simulink model "sampleModel1900"  (R2023a)
settings: Solver=VariableStepAuto  StartTime=0.0  StopTime=10.0  RelTol=1e-3
libraries: hdlsllib x2, simulink x1
settings Model: Creator=user1  LastModifiedBy=user1

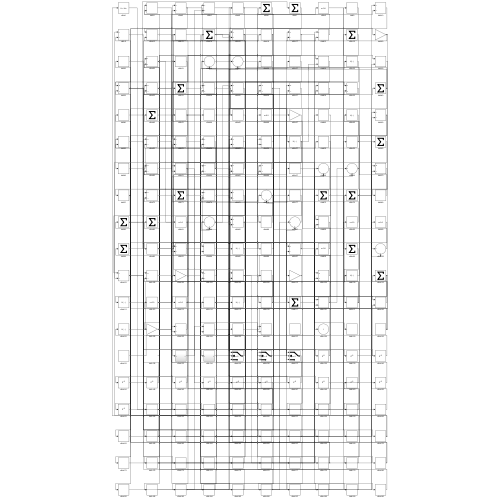
[thumbnail: Simulink's stored preview of the top-level diagram]
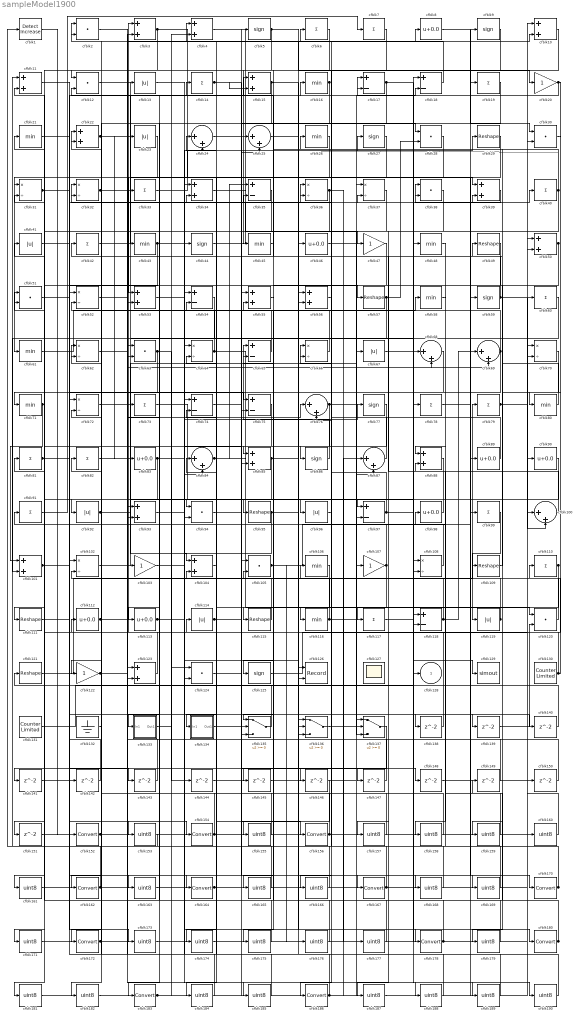
== system sampleModel1900 ==
  cfblk1 : simulink/Logic and Bit Operations/Detect Increase  vinit=0.0  OutDataTypeStr=boolean
      settings: LibrarySourceBlock=|
      | hdlsllib/Logic and Bit
      | Operations/Detect
      | Increase
  cfblk{3..4,10..11,15,22,34,39,50,53,55..56,85,88,93,101,104,123} (18 alike) : Sum
  cfblk{24..25,68..69,76,84,87,100} (8 alike) : Sum  Inputs=|++
  cfblk{31..32,36..37,52,62,64,66,70,72,102,108} (12 alike) : Product  Inputs=*/  RndMeth=Zero  SaturateOnIntegerOverflow=on
  cfblk{20,47,103,107,122} (5 alike) : Gain
  cfblk{2,12,28,30,38,51,63,94,105,120,124} (11 alike) : DotProduct  OutDataTypeStr=Inherit: Inherit via internal rule
  cfblk{16,21,26,43,45,48,58,61,71,80,106,116} (12 alike) : MinMax
  cfblk{29,49,57,95,109,111,115,121} (8 alike) : Reshape
  cfblk{6..7,14,19,33,40,42,60,73,78..79,81..82,91,99,110,117} (17 alike) : Sum  Inputs=+
  cfblk{8,46,83,89..90,98,112..113} (8 alike) : Bias  Bias=0.0  SaturateOnIntegerOverflow=off
  cfblk{13,23,41,67,92,96,114,119} (8 alike) : Abs  SaturateOnIntegerOverflow=off
  cfblk{17..18,35,54,65,74..75,97,118} (9 alike) : Sum  Inputs=+-
  cfblk{5,9,27,44,59,77,86,125} (8 alike) : Signum
  cfblk126 : Record  FileSettingsInternal="{\"entries\":[{\"content\":{\"excelSettings\":{\"content\":{},\"type\":\"Streamout.ExcelSettings\"}},\"type\":\"Streamout.FileSettingStorage\",\"uuid\":\"\"}],\"packageUris\":[\"http:\\/\\/schema.mathworks.com\\/mf0\\/streamout_blocks\\/R2020a\"],\"version\":\"1.0\"}"  Layout=[1 1]  SignalsInternal="{\"entries\":[{\"content\":{\"signals\":[{\"content\":{\"blockPath\":[],\"dimensions\":[1],\"domain\":\"\",\"lineColor\":\"#a2142f\",\"plots\":[1],\"port\":1,\"signalID\":4952,\"signalName\":\"XY Graph:1\"},\"type\":\"RecordBlkView.Signal\",\"uuid\":\"\"},{\"content\":{\"blockPath\":[],\"dimensions\":[1],\"domain\":\"\",\"lineColor\":\"#139fff\",\"plots\":[1],\"port\":2,\"signalID\":4955,\"signalName\":\"XY Graph:2\"},\"type\":\"RecordBlkView.Signal\",\"uuid\":\"\"}]},\"type\":\"RecordBlkView.InputSignals\",\"uuid\":\"\"}],\"packageUris\":[\"http:\\/\\/schema.mathworks.com\\/mf0\\/streamout_blocks\\/R2020a\"],\"version\":\"1.0\"}"  VisualizationBindings="{\"xyplotplugin\":{\"info\":[{\"series\":[{\"bindingParametersList\":[{\"parameter\":\"X-Axis\",\"signalID\":4952,\"signalName\":\"XY Graph:1\"},{\"parameter\":\"Y-Axis\",\"signalID\":4955,\"signalName\":\"XY Graph:2\"}],\"seriesID\":55809}],\"subplotID\":1}]}}"  CompatibilityTag=XY  st=-1
  cfblk127 : Scope
      settings: Floating=on
  cfblk129 : ToWorkspace  VariableName=simout  SaveFormat=Timeseries  SampleTime=-1
  cfblk130 : hdlsllib/Sources/Counter Limited  uplimit=7  tsamp=-1
  cfblk131 : hdlsllib/Sources/Counter Limited  uplimit=7  tsamp=-1
  cfblk132 : Ground
  cfblk133 : Subsystem
      settings: LibrarySourceBlock=|
      | hdlsllib/Ports &
      | Subsystems/Subsystem
  cfblk134 : Subsystem
      settings: LibrarySourceBlock=|
      | hdlsllib/Ports &
      | Subsystems/Subsystem
  cfblk135 : Switch  SaturateOnIntegerOverflow=off  InputSameDT=off
  cfblk136 : Switch  SaturateOnIntegerOverflow=off  InputSameDT=off
  cfblk137 : Switch  SaturateOnIntegerOverflow=off  InputSameDT=off
  cfblk{138..151} (14 alike) : Delay  SampleTime=1
  cfblk{152,154,156,162,164,167,170,172,178,180,183,186} (12 alike) : DataTypeConversion  SaturateOnIntegerOverflow=off  RndMeth=Floor
  cfblk{153,155,157..161,163,165..166,168..169,171,173..177,179,181..182,184..185,187..190} (27 alike) : DataTypeConversion  OutDataTypeStr=uint8  SaturateOnIntegerOverflow=off  RndMeth=Floor
  cfblk128 : Outport  VectorParamsAs1DForOutWhenUnconnected=off
  wires:
  cfblk108/1 -> cfblk91/1
  cfblk123/1 -> cfblk3/1
  cfblk58/1 -> cfblk117/1
  cfblk98/1 -> cfblk94/1
  cfblk84/1 -> cfblk120/1, cfblk35/1
  cfblk120/1 -> cfblk79/1
  cfblk86/1 -> cfblk65/1
  cfblk100/1 -> cfblk42/1
  cfblk73/1 -> cfblk96/1
  cfblk71/1 -> cfblk101/1, cfblk51/2
  cfblk91/1 -> cfblk7/1
  cfblk12/1 -> cfblk39/1
  cfblk32/1 -> cfblk104/1, cfblk75/1
  cfblk30/1 -> cfblk114/1
  cfblk110/1 -> cfblk118/2, cfblk157/1
  cfblk27/1 -> cfblk95/1
  cfblk118/1 -> cfblk84/1, cfblk69/1
  cfblk40/1 -> cfblk116/1, cfblk24/2, cfblk12/2
  cfblk42/1 -> cfblk16/1
  cfblk99/1 -> cfblk119/1
  cfblk82/1 -> cfblk154/1
  cfblk132/1 -> cfblk22/1
  cfblk74/1 -> cfblk156/1
  cfblk121/1 -> cfblk109/1
  cfblk54/1 -> cfblk183/1
  cfblk115/1 -> cfblk13/1
  cfblk26/1 -> cfblk134/1(In1)
  cfblk63/1 -> cfblk71/1, cfblk144/1
  cfblk105/1 -> cfblk9/1, cfblk176/1
  cfblk2/1 -> cfblk63/2
  cfblk75/1 -> cfblk133/1(In1)
  cfblk69/1 -> cfblk135/1, cfblk32/2
  cfblk18/1 -> cfblk6/1
  cfblk113/1 -> cfblk77/1, cfblk126/2
  cfblk44/1 -> cfblk38/1
  cfblk57/1 -> cfblk101/2, cfblk28/2, cfblk146/1
  cfblk17/1 -> cfblk128/1, cfblk33/1
  cfblk7/1 -> cfblk86/1
  cfblk85/1 -> cfblk46/1, cfblk93/2
  cfblk33/1 -> cfblk29/1
  cfblk5/1 -> cfblk20/1, cfblk151/1
  cfblk31/1 -> cfblk56/2, cfblk75/2, cfblk173/1
  cfblk80/1 -> cfblk26/1
  cfblk68/1 -> cfblk172/1
  cfblk4/1 -> cfblk47/1
  cfblk11/1 -> cfblk164/1
  cfblk102/1 -> cfblk34/1
  cfblk60/1 -> cfblk162/1
  cfblk117/1 -> cfblk48/1
  cfblk61/1 -> cfblk58/1
  cfblk133/1(Out1) -> cfblk124/1
  cfblk10/1 -> cfblk45/1
  cfblk15/1 -> cfblk92/1, cfblk57/1, cfblk125/1
  cfblk56/1 -> cfblk36/1
  cfblk122/1 -> cfblk40/1, cfblk69/2
  cfblk64/1 -> cfblk108/1, cfblk53/2
  cfblk23/1 -> cfblk61/1
  cfblk90/1 -> cfblk123/2
  cfblk22/1 -> cfblk118/1, cfblk83/1
  cfblk95/1 -> cfblk124/2, cfblk10/2
  cfblk1/1 -> cfblk152/1
  cfblk79/1 -> cfblk50/1, cfblk100/2
  cfblk119/1 -> cfblk102/2, cfblk73/1
  cfblk19/1 -> cfblk186/1
  cfblk39/1 -> cfblk38/2
  cfblk136/1 -> cfblk67/1
  cfblk35/1 -> cfblk135/2
  cfblk50/1 -> cfblk115/1, cfblk179/1
  cfblk16/1 -> cfblk113/1, cfblk182/1
  cfblk34/1 -> cfblk107/1
  cfblk37/1 -> cfblk135/3
  cfblk25/1 -> cfblk180/1
  cfblk131/1 -> cfblk108/2
  cfblk89/1 -> cfblk2/1
  cfblk101/1 -> cfblk51/1, cfblk143/1, cfblk163/1
  cfblk36/1 -> cfblk111/1, cfblk177/1
  cfblk65/1 -> cfblk22/2
  cfblk76/1 -> cfblk18/2, cfblk181/1
  cfblk3/1 -> cfblk99/1, cfblk12/1
  cfblk8/1 -> cfblk30/1
  cfblk97/1 -> cfblk129/1, cfblk66/1
  cfblk28/1 -> cfblk53/1
  cfblk46/1 -> cfblk137/1
  cfblk49/1 -> cfblk88/1
  cfblk114/1 -> cfblk136/2, cfblk148/1
  cfblk62/1 -> cfblk23/1
  cfblk111/1 -> cfblk137/2
  cfblk45/1 -> cfblk85/1
  cfblk41/1 -> cfblk17/1
  cfblk96/1 -> cfblk36/2
  cfblk20/1 -> cfblk17/2, cfblk80/1
  cfblk83/1 -> cfblk27/1, cfblk122/1
  cfblk43/1 -> cfblk84/2, cfblk35/2, cfblk171/1
  cfblk87/1 -> cfblk32/1
  cfblk125/1 -> cfblk10/1
  cfblk81/1 -> cfblk37/2, cfblk169/1
  cfblk9/1 -> cfblk31/1
  cfblk59/1 -> cfblk100/1, cfblk15/1
  cfblk51/1 -> cfblk137/3
  cfblk52/1 -> cfblk167/1
  cfblk116/1 -> cfblk39/2, cfblk62/1
  cfblk53/1 -> cfblk85/2
  cfblk66/1 -> cfblk24/1
  cfblk107/1 -> cfblk62/2, cfblk155/1
  cfblk78/1 -> cfblk170/1
  cfblk103/1 -> cfblk178/1
  cfblk109/1 -> cfblk49/1
  cfblk92/1 -> cfblk97/1, cfblk37/1
  cfblk112/1 -> cfblk76/1, cfblk8/1
  cfblk104/1 -> cfblk14/1
  cfblk14/1 -> cfblk15/2, cfblk139/1, cfblk140/1
  cfblk47/1 -> cfblk76/2
  cfblk135/1 -> cfblk41/1
  cfblk130/1 -> cfblk31/2, cfblk4/1, cfblk110/1
  cfblk24/1 -> cfblk28/1
  cfblk94/1 -> cfblk138/1
  cfblk138/1 -> cfblk34/2
  cfblk139/1 -> cfblk120/2
  cfblk140/1 -> cfblk104/2
  cfblk137/1 -> cfblk141/1
  cfblk21/1 -> cfblk142/1
  cfblk142/1 -> cfblk102/1
  cfblk143/1 -> cfblk93/1
  cfblk144/1 -> cfblk97/2
  cfblk29/1 -> cfblk145/1
  cfblk145/1 -> cfblk65/2
  cfblk124/1 -> cfblk147/1
  cfblk147/1 -> cfblk64/2
  cfblk148/1 -> cfblk50/2
  cfblk149/1 -> cfblk56/1
  cfblk150/1 -> cfblk123/1
  cfblk151/1 -> cfblk3/2
  cfblk152/1 -> cfblk136/1, cfblk90/1
  cfblk141/1 -> cfblk153/1
  cfblk153/1 -> cfblk1/1
  cfblk154/1 -> cfblk5/1, cfblk64/1
  cfblk155/1 -> cfblk82/1
  cfblk156/1 -> cfblk105/2, cfblk66/2, cfblk43/1, cfblk59/1
  cfblk157/1 -> cfblk74/1
  cfblk48/1 -> cfblk158/1
  cfblk158/1 -> cfblk74/2
  cfblk70/1 -> cfblk159/1
  cfblk159/1 -> cfblk98/1
  cfblk160/1 -> cfblk70/1
  cfblk88/1 -> cfblk161/1
  cfblk161/1 -> cfblk70/2
  cfblk162/1 -> cfblk94/2, cfblk21/1
  cfblk163/1 -> cfblk60/1
  cfblk164/1 -> cfblk136/3, cfblk89/1
  cfblk6/1 -> cfblk165/1
  cfblk165/1 -> cfblk11/1
  cfblk77/1 -> cfblk166/1
  cfblk166/1 -> cfblk11/2
  cfblk167/1 -> cfblk18/1, cfblk106/1
  cfblk134/1(Out1) -> cfblk168/1
  cfblk168/1 -> cfblk52/1
  cfblk169/1 -> cfblk52/2
  cfblk170/1 -> cfblk88/2, cfblk2/2
  cfblk171/1 -> cfblk78/1
  cfblk172/1 -> cfblk160/1, cfblk44/1
  cfblk173/1 -> cfblk68/1
  cfblk146/1 -> cfblk174/1
  cfblk174/1 -> cfblk68/2
  cfblk55/1 -> cfblk175/1
  cfblk175/1 -> cfblk112/1
  cfblk176/1 -> cfblk55/1
  cfblk177/1 -> cfblk55/2
  cfblk178/1 -> cfblk81/1, cfblk105/1
  cfblk179/1 -> cfblk103/1
  cfblk180/1 -> cfblk149/1, cfblk121/1
  cfblk181/1 -> cfblk25/1
  cfblk182/1 -> cfblk25/2
  cfblk183/1 -> cfblk150/1, cfblk4/2, cfblk87/2
  cfblk106/1 -> cfblk184/1
  cfblk184/1 -> cfblk54/1
  cfblk13/1 -> cfblk185/1
  cfblk185/1 -> cfblk54/2
  cfblk186/1 -> cfblk126/1, cfblk30/2, cfblk87/1
  cfblk38/1 -> cfblk187/1
  cfblk187/1 -> cfblk19/1
  cfblk72/1 -> cfblk188/1
  cfblk188/1 -> cfblk63/1
  cfblk93/1 -> cfblk189/1
  cfblk189/1 -> cfblk72/1
  cfblk67/1 -> cfblk190/1
  cfblk190/1 -> cfblk72/2

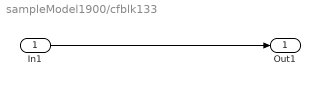
== system sampleModel1900/cfblk133 ==
  In1 : Inport
  Out1 : Outport
  wires:
  In1/1 -> Out1/1

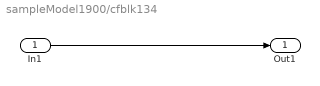
== system sampleModel1900/cfblk134 ==
  In1 : Inport
  Out1 : Outport
  wires:
  In1/1 -> Out1/1
